simulink library "IGRF"  (R2014b)
settings: Solver=ode45  StartTime=0.0  StopTime=10.0  RelTol=1e-3
undefined symbols (not defined in the file or in its folder): ConfParam
libraries: J2000toGeoc x1
settings Model: Creator=Hp  LastModifiedBy=Hp

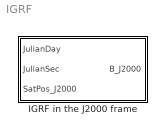
== system IGRF ==
  IGRF in the J2000 frame : Subsystem

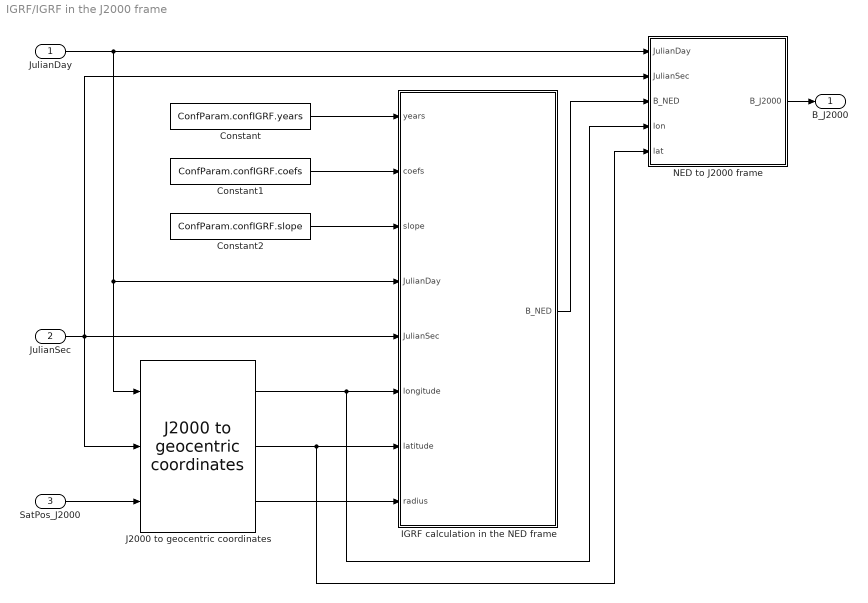
== system IGRF/IGRF in the J2000 frame ==
  JulianDay : Inport
  JulianSec : Inport  Port=2
  SatPos_J2000 : Inport  Port=3
  Constant : Constant  Value=ConfParam.confIGRF.years
  Constant1 : Constant  Value=ConfParam.confIGRF.coefs
  Constant2 : Constant  Value=ConfParam.confIGRF.slope
  IGRF calculation in the NED frame : MATLAB Function  TreatAsAtomicUnit=on
  J2000 to geocentric coordinates : J2000toGeoc/J2000 to geocentric coordinates
  NED to J2000 frame : Subsystem
  B_J2000 : Outport
  wires:
  J2000 to geocentric coordinates/2 -> NED to J2000 frame/5(lat), IGRF calculation in the NED frame/7(latitude)
  SatPos_J2000/1 -> J2000 to geocentric coordinates/3
  J2000 to geocentric coordinates/1 -> NED to J2000 frame/4(lon), IGRF calculation in the NED frame/6(longitude)
  JulianSec/1 -> J2000 to geocentric coordinates/2, IGRF calculation in the NED frame/5(JulianSec), NED to J2000 frame/2(JulianSec)
  JulianDay/1 -> J2000 to geocentric coordinates/1, IGRF calculation in the NED frame/4(JulianDay), NED to J2000 frame/1(JulianDay)
  NED to J2000 frame/1(B_J2000) -> B_J2000/1
  Constant/1 -> IGRF calculation in the NED frame/1(years)
  Constant1/1 -> IGRF calculation in the NED frame/2(coefs)
  Constant2/1 -> IGRF calculation in the NED frame/3(slope)
  IGRF calculation in the NED frame/1(B_NED) -> NED to J2000 frame/3(B_NED)
  J2000 to geocentric coordinates/3 -> IGRF calculation in the NED frame/8(radius)

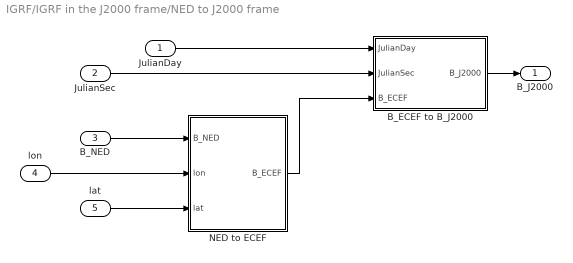
== system IGRF/IGRF in the J2000 frame/NED to J2000 frame ==
  JulianDay : Inport
  JulianSec : Inport  Port=2
  B_NED : Inport  Port=3
  lon : Inport  Port=4
  lat : Inport  Port=5
  B_ECEF to B_J2000 : Subsystem
  NED to ECEF : Subsystem
  B_J2000 : Outport
  wires:
  JulianSec/1 -> B_ECEF to B_J2000/2(JulianSec)
  NED to ECEF/1(B_ECEF) -> B_ECEF to B_J2000/3(B_ECEF)
  B_ECEF to B_J2000/1(B_J2000) -> B_J2000/1
  B_NED/1 -> NED to ECEF/1(B_NED)
  JulianDay/1 -> B_ECEF to B_J2000/1(JulianDay)
  lon/1 -> NED to ECEF/2(lon)
  lat/1 -> NED to ECEF/3(lat)

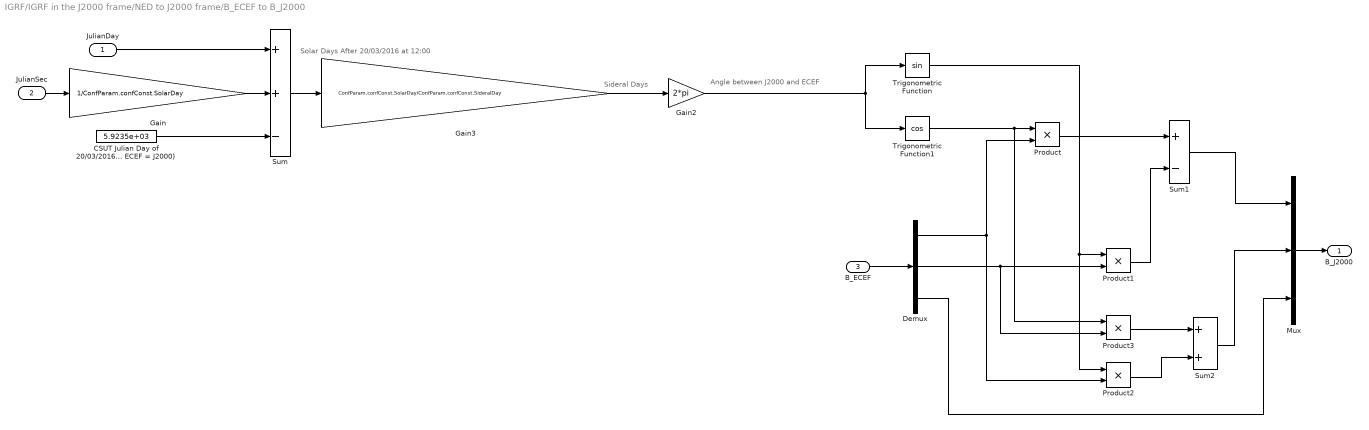
== system IGRF/IGRF in the J2000 frame/NED to J2000 frame/B_ECEF to B_J2000 ==
  note: Angle between J2000 and ECEF
  note: Sideral Days
  note: Solar Days After 20/03/2016 at 12:00
  JulianDay : Inport
  JulianSec : Inport  Port=2
  B_ECEF : Inport  Port=3
  CSUT Julian Day of 20/03/2016 at 12:00 UTC (moment in which ECEF = J2000) : Constant  Value=5.9235e+03
  Demux : Demux  Outputs=3
  Gain : Gain  Gain=1/ConfParam.confConst.SolarDay
  Gain2 : Gain  Gain=2*pi
  Gain3 : Gain  Gain=ConfParam.confConst.SolarDay/ConfParam.confConst.SideralDay
  Mux : Mux  Inputs=3
  Product{,1..3} (4 alike) : Product
  Sum : Sum  Inputs=++-
  Sum1 : Sum  Inputs=+-
  Sum2 : Sum
  Trigonometric Function : Trigonometry
  Trigonometric Function1 : Trigonometry  Operator=cos
  B_J2000 : Outport
  wires:
  JulianDay/1 -> Sum/1
  JulianSec/1 -> Gain/1
  Gain/1 -> Sum/2
  CSUT Julian Day of 20/03/2016 at 12:00 UTC (moment in which ECEF = J2000)/1 -> Sum/3
  Sum/1 -> Gain3/1
  Gain3/1 -> Gain2/1
  B_ECEF/1 -> Demux/1
  Gain2/1 -> Trigonometric Function1/1, Trigonometric Function/1
  Trigonometric Function1/1 -> Product3/1, Product/1
  Demux/1 -> Product2/2, Product/2
  Product/1 -> Sum1/1
  Trigonometric Function/1 -> Product2/1, Product1/1
  Demux/2 -> Product3/2, Product1/2
  Product1/1 -> Sum1/2
  Sum1/1 -> Mux/1
  Product2/1 -> Sum2/2
  Product3/1 -> Sum2/1
  Sum2/1 -> Mux/2
  Mux/1 -> B_J2000/1
  Demux/3 -> Mux/3

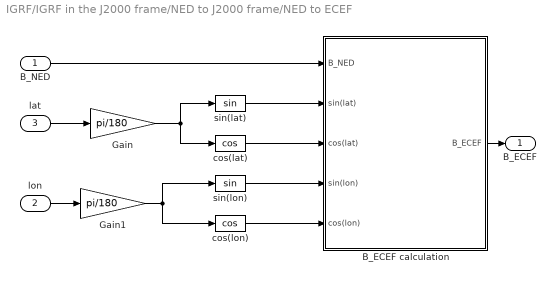
== system IGRF/IGRF in the J2000 frame/NED to J2000 frame/NED to ECEF ==
  B_NED : Inport
  lon : Inport  Port=2
  lat : Inport  Port=3
  B_ECEF calculation : Subsystem
  Gain : Gain  Gain=pi/180
  Gain1 : Gain  Gain=pi/180
  cos(lat) : Trigonometry  Operator=cos
  cos(lon) : Trigonometry  Operator=cos
  sin(lat) : Trigonometry
  sin(lon) : Trigonometry
  B_ECEF : Outport
  wires:
  cos(lon)/1 -> B_ECEF calculation/5(cos(lon))
  sin(lon)/1 -> B_ECEF calculation/4(sin(lon))
  cos(lat)/1 -> B_ECEF calculation/3(cos(lat))
  sin(lat)/1 -> B_ECEF calculation/2(sin(lat))
  B_NED/1 -> B_ECEF calculation/1(B_NED)
  Gain/1 -> cos(lat)/1, sin(lat)/1
  Gain1/1 -> sin(lon)/1, cos(lon)/1
  lon/1 -> Gain1/1
  B_ECEF calculation/1(B_ECEF) -> B_ECEF/1
  lat/1 -> Gain/1

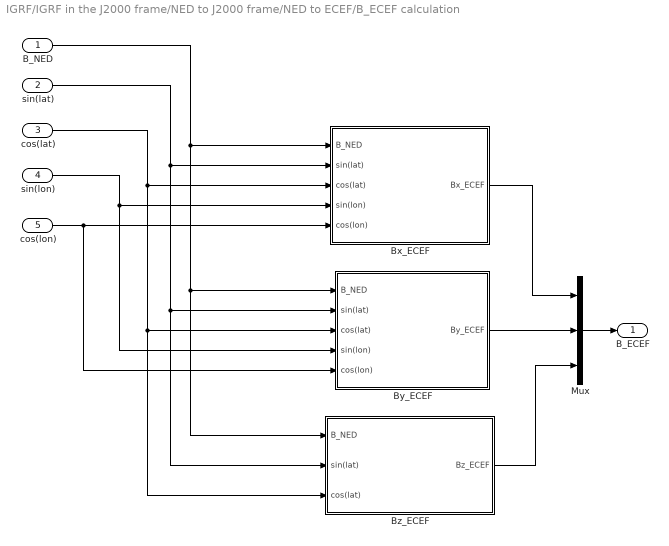
== system IGRF/IGRF in the J2000 frame/NED to J2000 frame/NED to ECEF/B_ECEF calculation ==
  B_NED : Inport
  sin(lat) : Inport  Port=2
  cos(lat) : Inport  Port=3
  sin(lon) : Inport  Port=4
  cos(lon) : Inport  Port=5
  Bx_ECEF : Subsystem
  By_ECEF : Subsystem
  Bz_ECEF : Subsystem
  Mux : Mux  Inputs=3
  B_ECEF : Outport
  wires:
  Mux/1 -> B_ECEF/1
  Bz_ECEF/1(Bz_ECEF) -> Mux/3
  Bx_ECEF/1(Bx_ECEF) -> Mux/1
  By_ECEF/1(By_ECEF) -> Mux/2
  sin(lat)/1 -> Bx_ECEF/2(sin(lat)), By_ECEF/2(sin(lat)), Bz_ECEF/2(sin(lat))
  B_NED/1 -> Bx_ECEF/1(B_NED), By_ECEF/1(B_NED), Bz_ECEF/1(B_NED)
  cos(lon)/1 -> Bx_ECEF/5(cos(lon)), By_ECEF/5(cos(lon))
  sin(lon)/1 -> Bx_ECEF/4(sin(lon)), By_ECEF/4(sin(lon))
  cos(lat)/1 -> Bx_ECEF/3(cos(lat)), By_ECEF/3(cos(lat)), Bz_ECEF/3(cos(lat))

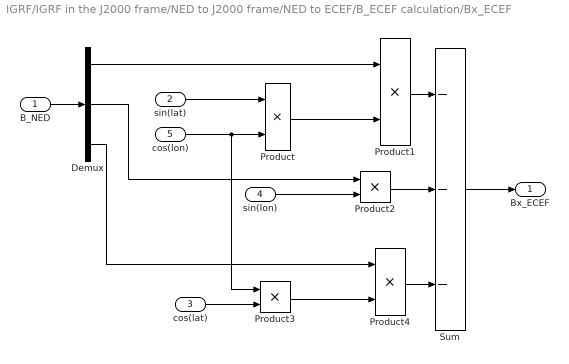
== system IGRF/IGRF in the J2000 frame/NED to J2000 frame/NED to ECEF/B_ECEF calculation/Bx_ECEF ==
  B_NED : Inport
  sin(lat) : Inport  Port=2
  cos(lat) : Inport  Port=3
  sin(lon) : Inport  Port=4
  cos(lon) : Inport  Port=5
  Demux : Demux  Outputs=3
  Product{,1..4} (5 alike) : Product
  Sum : Sum  Inputs=---
  Bx_ECEF : Outport
  wires:
  B_NED/1 -> Demux/1
  Product3/1 -> Product4/2
  Product2/1 -> Sum/2
  Product4/1 -> Sum/3
  Product1/1 -> Sum/1
  Sum/1 -> Bx_ECEF/1
  cos(lat)/1 -> Product3/2
  Demux/3 -> Product4/1
  sin(lon)/1 -> Product2/2
  Demux/1 -> Product1/1
  sin(lat)/1 -> Product/1
  Demux/2 -> Product2/1
  Product/1 -> Product1/2
  cos(lon)/1 -> Product/2, Product3/1

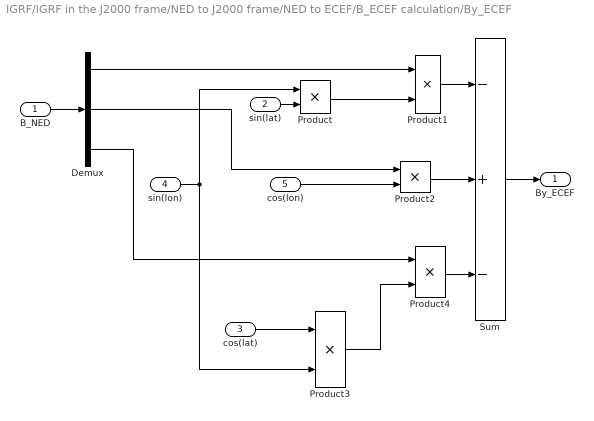
== system IGRF/IGRF in the J2000 frame/NED to J2000 frame/NED to ECEF/B_ECEF calculation/By_ECEF ==
  B_NED : Inport
  sin(lat) : Inport  Port=2
  cos(lat) : Inport  Port=3
  sin(lon) : Inport  Port=4
  cos(lon) : Inport  Port=5
  Demux : Demux  Outputs=3
  Product{,1..4} (5 alike) : Product
  Sum : Sum  Inputs=-+-
  By_ECEF : Outport
  wires:
  B_NED/1 -> Demux/1
  Product3/1 -> Product4/2
  Product2/1 -> Sum/2
  Product4/1 -> Sum/3
  Product1/1 -> Sum/1
  Sum/1 -> By_ECEF/1
  cos(lat)/1 -> Product3/1
  Demux/3 -> Product4/1
  sin(lon)/1 -> Product3/2, Product/1
  Demux/1 -> Product1/1
  sin(lat)/1 -> Product/2
  Demux/2 -> Product2/1
  Product/1 -> Product1/2
  cos(lon)/1 -> Product2/2

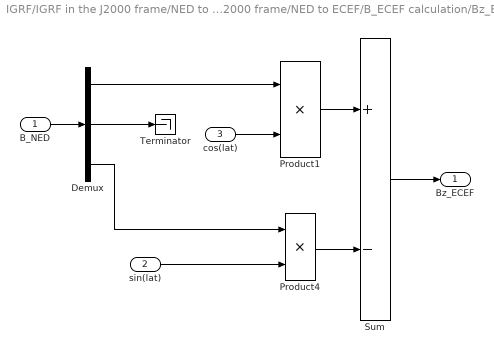
== system IGRF/IGRF in the J2000 frame/NED to J2000 frame/NED to ECEF/B_ECEF calculation/Bz_ECEF ==
  B_NED : Inport
  sin(lat) : Inport  Port=2
  cos(lat) : Inport  Port=3
  Demux : Demux  Outputs=3
  Product1 : Product
  Product4 : Product
  Sum : Sum  Inputs=+-
  Terminator : Terminator
  Bz_ECEF : Outport
  wires:
  sin(lat)/1 -> Product4/2
  cos(lat)/1 -> Product1/2
  Demux/2 -> Terminator/1
  B_NED/1 -> Demux/1
  Product4/1 -> Sum/2
  Product1/1 -> Sum/1
  Sum/1 -> Bz_ECEF/1
  Demux/3 -> Product4/1
  Demux/1 -> Product1/1

== matlab function IGRF/IGRF in the J2000 frame/IGRF calculation in the NED frame ==
  data: years input; coefs input; slope input; JulianDay input; JulianSec input; longitude input; B_NED output; latitude input; radius input
function B_NED = igrf(years, coefs, slope, JulianDay, JulianSec, longitude, latitude, radius)

% IGRF Earth's magnetic field from IGRF model.
%  
% Calculates the components of the Earth's magnetic field using the
% International Geomagnetic Reference Field (IGRF) model. 
% 
% Note that the other parameters the IGRF gives can be computed from BX,
% BY, and BZ as:
% 
%   Horizonal intensity: hypot(BX, BY) (i.e., sqrt(BX.^2 + BY.^2) )
%   Total intensity: hypot(BX, hypot(BY, BZ))
%   Declination: atan2(BY, BX)
%   Inclination: atan(BZ./hypot(BX, BY))
% 
% This function relies on having the file igrfcoefs.mat in the MATLAB
% path to function properly when a time is input.
% 
% The IGRF is a spherical harmonic expansion of the Earth's internal
% magnetic field. Currently, the IGRF model is valid between the years 1900
% and 2015. See the health warning for the IGRF model here:
% http://www.ngdc.noaa.gov/IAGA/vmod/igrfhw.html
% 
% Reference:
% International Association of Geomagnetism and Aeronomy, Working Group 
% V-MOD (2010), International Geomagnetic Reference Field: the eleventh
% generation, _Geophys. J. Int._, _183_(3), 1216-1230, 
% doi:10.1111/j.1365-246X.2010.04804.x.
% 
% Inputs:
%   -JULIANDAY: julian day in which this function calculates the magnetic
%   field of the Earth [integer].
%   -JULIANSEC: Number of seconds passed in the day JULIANDAY at the moment
%   in which this function calculates the magnetic field of the Earth
%   [double].
%   -LATITUDE: Geocentric latitude in degrees.
%   -LONGITUDE: Geocentric longitude in degrees.
%   -RADIUS: The radius in m from the center of the Earth to the satellite
%   center of gravity.
% 
% Outputs:
%   -B_NED: The magnetic field in teslas (T) in the J2000 frame 
% 
% See also: LOADIGRFCOEFS, DATENUM, IGRF11MAGM.

radius=radius/1000; %radius in km

% Fundamental constant.
Rearth_km = 6371.2;

time = JulianDay+JulianSec/86400; % Julian Day (decimal)

% Time convention of Matlab serial date number
time = time+730486;

% Check that the input coordinates are scalars.
if ~isscalar(latitude) || ~isscalar(longitude) || ~isscalar(radius)
    error('igrf1:inputNotScalar', ...
        'The input coordinates must be scalars.');
end

%%% SPHERICAL COORDINATE CONVERSION %%%
% Convert the latitude, longitude, and radius coordinates input into
% spherical coordinates r (radius), theta (inclination angle from +z axis),
% and phi (azimuth angle from +x axis).
% We want cos(theta) and sin(theta) rather than theta itself.
costheta = cos((90 - latitude)*pi/180);
sintheta = sin((90 - latitude)*pi/180);

r = radius;

% Convert longitude to radians.
phi = longitude*pi/180;

%%% GET PROPER IGRF COEFFICIENTS %%%
% Thie next line lets Simulink start the loadigrfcoefs_PILIA function
coder.extrinsic('loadigrfcoefs_PILIA'); 

% Before launching the loadigrfcoefs_PILIA function from the Simulink
% model, we also have to define the dimensions of gh
gh = zeros(195,1); % we have 195 coefficients for our IGRF model

gh = loadigrfcoefs_PILIA(time, years, coefs, slope);
nmax = sqrt(length(gh) + 1) - 1;

% We need cos(m*phi) and sin(m*phi) multiple times, so precalculate into a
% vector here:
cosphi = cos((1:nmax)*phi);
sinphi = sin((1:nmax)*phi);

Pmax = (nmax+1)*(nmax+2)/2;

%%% BEGIN MAGNETIC FIELD CALCULATION %%%
% Initialize variables used in for loop below.
Br = 0; Bt = 0; Bp = 0;
 P = zeros(1, Pmax);  P(1) = 1;  P(3) = sintheta;
dP = zeros(1, Pmax); dP(1) = 0; dP(3) = costheta;

% For this initial condition, the first if will result in n = 1, m = 0.
m = 1; n = 0; coefindex = 1;

a_r = (Rearth_km/r)^2;

% Increment through all the n's and m's. gh will be a vector with g
% followed by h for incrementing through n and m except when h would be
% redundant (i.e., when m = 0).
for Pindex = 2:Pmax
    
    % Increment to the next n when m becomes larger than n.
    if n < m
        m = 0;
        n = n + 1;
        a_r = a_r*(Rearth_km/r); % We need (Rearth_km./r)^(n+2)
    end
    
    % Calculate P and dP. They are given recursively according to:
    % 
    % P(0, 0) = 1, P(1, 1) = sin(theta) <- Specified above
    % P(n, n) = sqrt(1 - 1/(2n))*sin(theta)*P(n-1, n-1)
    % P(n, m) = (2n - 1)/sqrt(n^2 - m^2)*cos(theta)*P(n-1, m) -
    %     sqrt(((n-1)^2 - m^2) / (n^2 - m^2)) * P(n-2, m)
    % 
    % dP(0, 0) = 0, dP(1, 1) = cos(theta) <- Specified above
    % dP(n, n) = sqrt(1 - 1/(2n))*(sin(theta)*dP(n-1, n-1) +
    %     cos(theta)*P(n-1, n-1))
    % dP(n, m) = (2n - 1)/sqrt(n^2 - m^2)*(cos(theta)*dP(n-1, m) -
    %     sin(theta)*P(n-1, m)) - sqrt(((n-1)^2 - m^2)/(n^2 - m^2))*
    %     dP(n-2, m)
    if m < n && Pindex ~= 3 % (Pindex=3 is n=1, m=1, initial cond. above)
        last1n = Pindex - n;
        last2n = Pindex - 2*n + 1;
        P(Pindex) = (2*n - 1)/sqrt(n^2 - m^2)*costheta*P(last1n) - ...
            sqrt(((n-1)^2 - m^2) / (n^2 - m^2)) * P(last2n);
        dP(Pindex) = (2*n - 1)/sqrt(n^2 - m^2)*(costheta*dP(last1n) - ...
            sintheta*P(last1n)) - sqrt(((n-1)^2 - m^2) / (n^2 - m^2)) * ...
            dP(last2n);
    elseif Pindex ~= 3
        lastn = Pindex - n - 1;
        P(Pindex) = sqrt(1 - 1/(2*m))*sintheta*P(lastn);
        dP(Pindex) = sqrt(1 - 1/(2*m))*(sintheta*dP(lastn) + ...
            costheta*P(lastn));
    end
    
    % Calculate the magnetic field components as a running sum. Find
    % explicit expressions for these in Global Earth Physics: a Handbook of
    % Physical Constants by Thomas J. Aherns (1995), pg. 49. Link:
    % http://books.google.com/books?id=aqjU_NHyre4C&lpg=PP1&dq=Global%20
    % earth%20physics%3A%20a%20handbook%20of%20physical%20constants&pg=PA49
    % #v=onepage&q&f=false
    % (except equation 6 is missing a required 1/sin(theta) and m; correct
    % equations on page 5 (equations 3a-3c) of:
    % http://hanspeterschaub.info/Papers/UnderGradStudents/
    % MagneticField.pdf)
    if m == 0 % Implies h = 0, so only coefficient in gh is g
        coef = a_r*gh(coefindex); %*cos(0*phi) = 1
        Br = Br + (n+1)*coef*P(Pindex);
        Bt = Bt - coef*dP(Pindex);
        % Bp is 0 for m = 0.
        coefindex = coefindex + 1; % Only need to skip over g this time.
    else
        coef = a_r*(gh(coefindex)*cosphi(m) + gh(coefindex+1)*sinphi(m));
        Br = Br + (n+1)*coef*P(Pindex);
        Bt = Bt - coef*dP(Pindex);
        if sintheta == 0 % Use different formula when dividing by 0.
            Bp = Bp - costheta*a_r*(-gh(coefindex)*sinphi(m) + ...
                gh(coefindex+1)*cosphi(m))*dP(Pindex);
        else
            Bp = Bp - 1/sintheta*a_r*m*(-gh(coefindex)*sinphi(m) + ...
                gh(coefindex+1)*cosphi(m))*P(Pindex);
        end
        coefindex = coefindex + 2; % Skip over g and h this time.
    end
    
    % Increment m.
    m = m + 1;
    
end

% % Convert from spherical to (x,y,z) = (North,East,Down).
Bx_NED = -Bt*1e-9; % Bt == B_theta is towards the south
By_NED = Bp*1e-9;
Bz_NED = -Br*1e-9;

B_NED=[Bx_NED; By_NED; Bz_NED];

end
